simulink model "Sistema"  (R2020a)
settings: Solver=VariableStepAuto  StartTime=0.0  StopTime=10.0  RelTol=1e-3
libraries: cstblocks x6
settings Model: Creator=celim  LastModifiedBy=celim

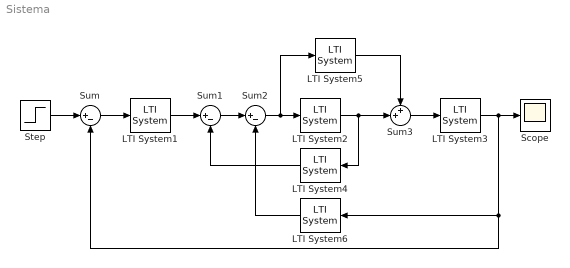
== system Sistema ==
  LTI System1 : cstblocks/LTI System  sys=G1  IC=[]
  LTI System2 : cstblocks/LTI System  sys=G2  IC=[]
  LTI System3 : cstblocks/LTI System  sys=G3  IC=[]
  LTI System4 : cstblocks/LTI System  sys=H2  IC=[]
  LTI System5 : cstblocks/LTI System  sys=H1  IC=[]
  LTI System6 : cstblocks/LTI System  sys=H3  IC=[]
  Scope : Scope
  Step : Step  SampleTime=0
  Sum : Sum  Inputs=|+-
  Sum1 : Sum  Inputs=|+-
  Sum2 : Sum  Inputs=|+-
  Sum3 : Sum  Inputs=++|
  wires:
  Step/1 -> Sum/1
  Sum/1 -> LTI System1/1
  LTI System1/1 -> Sum1/1
  Sum1/1 -> Sum2/1
  Sum2/1 -> LTI System5/1, LTI System2/1
  LTI System5/1 -> Sum3/1
  LTI System2/1 -> LTI System4/1, Sum3/2
  Sum3/1 -> LTI System3/1
  LTI System4/1 -> Sum1/2
  LTI System3/1 -> Sum/2, LTI System6/1, Scope/1
  LTI System6/1 -> Sum2/2
